simulink model "Sky_Sailor_Simulation"  (Simulink 8.3)
settings: Solver=ode3  StartTime=0.0  StopTime=20  FixedStep=0.05  RelTol=1e-3
libraries: simulink x1
settings Model: Creator=lestefan  LastModifiedBy=daniel
settings DataIOCC: ExternalInput=lw
settings OptimizationCC: ExpressionDepthLimit=2147483647  InitFltsAndDblsToZero=on
settings DebuggingCC: SaveWithParameterizedLinksMsg=none  SignalResolutionControl=TryResolveAllWithWarning  MultiTaskDSMMsg=warning  MultiTaskCondExecSysMsg=none  FcnCallInpInsideContextMsg=UseLocalSettings
settings SFSimCC: SimParseCustomCode=off
settings RTWCC: IncludeERTFirstTime=on
settings GRTTargetCC: TargetFcnLib=ansi_tfl_tmw.mat

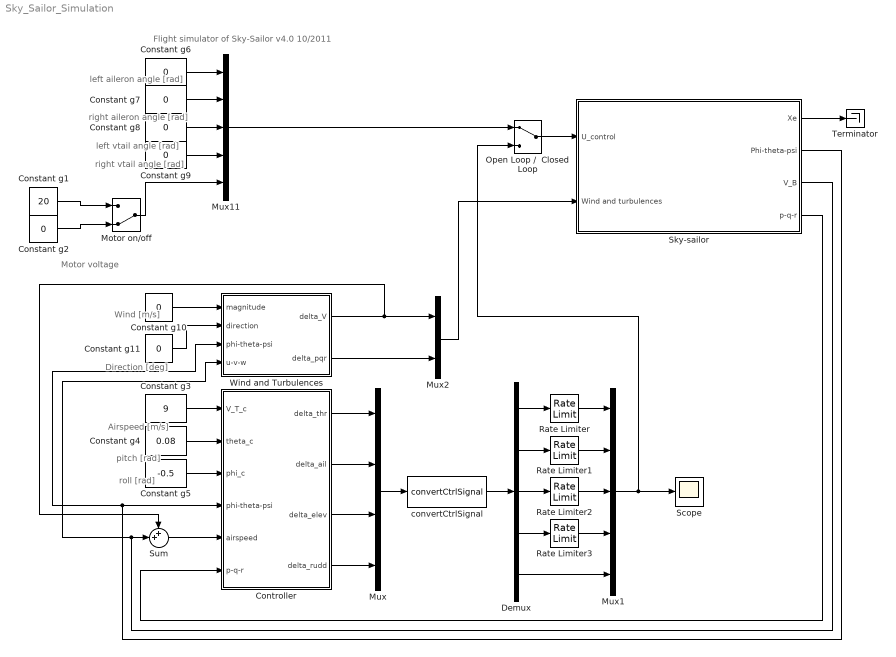
== system Sky_Sailor_Simulation ==
  note: Flight simulator of Sky-Sailor v4.0 10/2011
  note: left aileron angle [rad]
  note: right aileron angle [rad]
  note: left vtail angle [rad]
  note: right vtail angle [rad]
  note: Motor voltage
  note: Airspeed [m/s]
  note: pitch [rad]
  note: roll [rad]
  note: Wind [m/s]
  note: Direction [deg]
  Constant g1 : Constant  Value=20
  Constant g{2,6..11} (7 alike) : Constant  Value=0
  Constant g3 : Constant  Value=9
  Constant g4 : Constant  Value=0.08
  Constant g5 : Constant  Value=-0.5
  Controller : Subsystem
  Demux : Demux  Outputs=5
  Motor on/off : ManualSwitch  CurrentSetting=0
  Mux : Mux
  Mux1 : Mux  Inputs=5
  Mux11 : Mux  Inputs=5
  Mux2 : Mux  Inputs=2
  Open Loop /  Closed Loop : ManualSwitch
  Rate Limiter{,1..3} (4 alike) : RateLimiter  RisingSlewLimit=pi  FallingSlewLimit=-pi  SampleTimeMode=inherited
  Scope : Scope
      settings: YMin=-2.5  YMax=30  SaveName=ScopeData7
  Sky-sailor : Subsystem
  Sum : Sum  Inputs=++|
  Terminator : Terminator
  Wind and Turbulences : Subsystem
  convertCtrlSignal : MATLABFcn  MATLABFcn=convertCtrlSignal  OutputDimensions=5  OutputSignalType=real
  wires:
  Constant g6/1 -> Mux11/1
  Constant g7/1 -> Mux11/2
  Constant g8/1 -> Mux11/3
  Constant g9/1 -> Mux11/4
  Motor on/off/1 -> Mux11/5
  Sky-sailor/1(Xe) -> Terminator/1
  Constant g1/1 -> Motor on/off/1
  Constant g2/1 -> Motor on/off/2
  Constant g3/1 -> Controller/1(V_T_c)
  Constant g4/1 -> Controller/2(theta_c)
  Constant g5/1 -> Controller/3(phi_c)
  Mux11/1 -> Open Loop /  Closed Loop/1
  Open Loop /  Closed Loop/1 -> Sky-sailor/1(U_control)
  Mux1/1 -> Open Loop /  Closed Loop/2, Scope/1
  Sky-sailor/2(Phi-theta-psi) -> Controller/4(phi-theta-psi), Wind and Turbulences/3(phi-theta-psi)
  Sky-sailor/4(p-q-r) -> Controller/6(p-q-r)
  Controller/1(delta_thr) -> Mux/1
  Controller/2(delta_ail) -> Mux/2
  Controller/4(delta_rudd) -> Mux/4
  Demux/1 -> Rate Limiter/1
  Demux/2 -> Rate Limiter1/1
  Demux/3 -> Rate Limiter2/1
  Demux/4 -> Rate Limiter3/1
  Demux/5 -> Mux1/5
  Controller/3(delta_elev) -> Mux/3
  Rate Limiter/1 -> Mux1/1
  Rate Limiter1/1 -> Mux1/2
  Rate Limiter2/1 -> Mux1/3
  Rate Limiter3/1 -> Mux1/4
  Constant g10/1 -> Wind and Turbulences/1(magnitude)
  Sky-sailor/3(V_B) -> Sum/2, Wind and Turbulences/4(u-v-w)
  Sum/1 -> Controller/5(airspeed)
  Mux2/1 -> Sky-sailor/2(Wind and turbulences)
  Wind and Turbulences/1(delta_V) -> Mux2/1, Sum/1
  Wind and Turbulences/2(delta_pqr) -> Mux2/2
  Constant g11/1 -> Wind and Turbulences/2(direction)
  Mux/1 -> convertCtrlSignal/1
  convertCtrlSignal/1 -> Demux/1

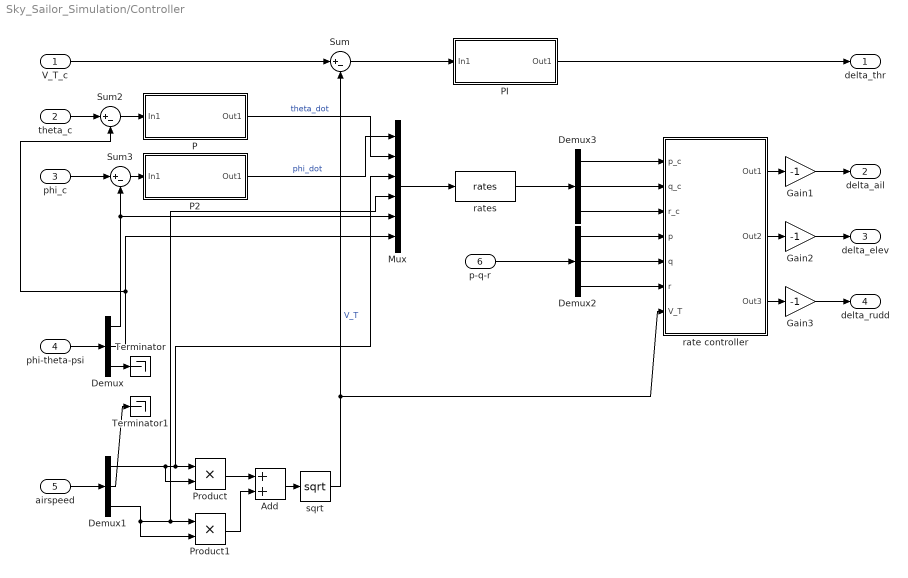
== system Sky_Sailor_Simulation/Controller ==
  V_T_c : Inport
  theta_c : Inport  Port=2
  phi_c : Inport  Port=3
  phi-theta-psi : Inport  Port=4
  airspeed : Inport  Port=5
  p-q-r : Inport  Port=6
  Add : Sum
  Demux{,1..3} (4 alike) : Demux  Outputs=3
  Gain1 : Gain  Gain=-1
  Gain2 : Gain  Gain=-1
  Gain3 : Gain  Gain=-1
  Mux : Mux  Inputs=6
  P : Subsystem
  P2 : Subsystem
  PI : Subsystem
  Product : Product  RndMeth=Zero
  Product1 : Product  RndMeth=Zero
  Sum : Sum  Inputs=|+-
  Sum2 : Sum  Inputs=|+-
  Sum3 : Sum  Inputs=|+-
  Terminator : Terminator
  Terminator1 : Terminator
  rate controller : Subsystem
  rates : MATLABFcn  MATLABFcn=rates  OutputDimensions=3  Output1D=off
  sqrt : Math  Operator=sqrt  SaturateOnIntegerOverflow=on
  delta_thr : Outport
  delta_ail : Outport  Port=2
  delta_elev : Outport  Port=3
  delta_rudd : Outport  Port=4
  wires:
  PI/1(Out1) -> delta_thr/1
  Gain1/1 -> delta_ail/1
  Gain2/1 -> delta_elev/1
  Gain3/1 -> delta_rudd/1
  phi-theta-psi/1 -> Demux/1
  airspeed/1 -> Demux1/1
  V_T_c/1 -> Sum/1
  Sum/1 -> PI/1(In1)
  Demux1/1 -> Product/1, Product/2, Mux/3
  Product/1 -> Add/1
  p-q-r/1 -> Demux2/1
  Product1/1 -> Add/2
  Add/1 -> sqrt/1
  sqrt/1 -> Sum/2, rate controller/7(V_T)  "V_T"
  Demux1/3 -> Product1/2, Product1/1, Mux/4
  Demux/1 -> Sum3/2, Mux/5
  Demux/2 -> Mux/6, Sum2/2
  theta_c/1 -> Sum2/1
  Sum2/1 -> P/1(In1)
  phi_c/1 -> Sum3/1
  Sum3/1 -> P2/1(In1)
  rate controller/1(Out1) -> Gain1/1
  rate controller/2(Out2) -> Gain2/1
  rate controller/3(Out3) -> Gain3/1
  Demux2/1 -> rate controller/4(p)
  Demux2/2 -> rate controller/5(q)
  Demux2/3 -> rate controller/6(r)
  Demux/3 -> Terminator/1
  Mux/1 -> rates/1
  P2/1(Out1) -> Mux/1  "phi_dot"
  P/1(Out1) -> Mux/2  "theta_dot"
  Demux1/2 -> Terminator1/1
  rates/1 -> Demux3/1
  Demux3/1 -> rate controller/1(p_c)
  Demux3/2 -> rate controller/2(q_c)
  Demux3/3 -> rate controller/3(r_c)

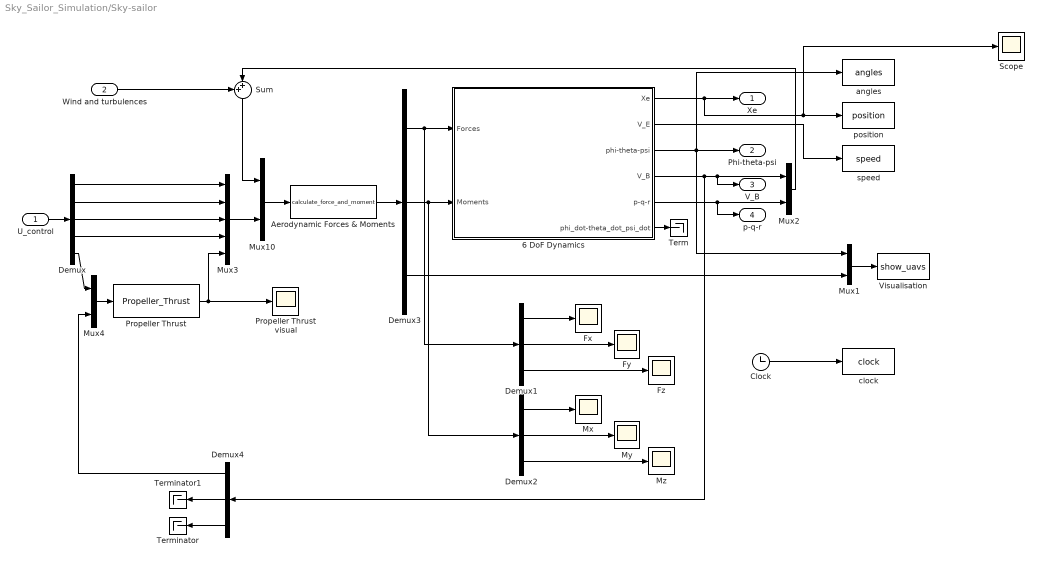
== system Sky_Sailor_Simulation/Sky-sailor ==
  U_control : Inport
  Wind and turbulences : Inport  Port=2
  "6 DoF Dynamics " : Subsystem
  Aerodynamic Forces & Moments : MATLABFcn  MATLABFcn=calculate_force_and_moment  OutputDimensions=7
  Clock : Clock
  Demux : Demux  Outputs=5
  Demux{1..4} (4 alike) : Demux  Outputs=3
  Fx : Scope
      settings: YMin=-0.58075  YMax=-0.57875
  Fy : Scope
      settings: YMin=-7e-016  YMax=4e-016
  Fz : Scope
      settings: YMin=-25.5725  YMax=-25.5325  SaveName=ScopeData2
  Mux{1..2,4,10} (4 alike) : Mux  Inputs=2
  Mux3 : Mux  Inputs=5
  Mx : Scope
      settings: YMin=-5e-015  YMax=5e-015  SaveName=ScopeData4
  My : Scope
      settings: YMin=-0.00025  YMax=0.0004  SaveName=ScopeData5
  Mz : Scope
      settings: YMin=-1.25e-016  YMax=1.75e-016  SaveName=ScopeData6
  Propeller Thrust : MATLABFcn  MATLABFcn=Propeller_Thrust  OutputDimensions=1
  Propeller Thrust visual : Scope
      settings: YMin=1.175  YMax=1.193  SaveName=ScopeData8
  Scope : Scope
      settings: SaveName=ScopeData3
  Sum : Sum  Inputs=++|
  Term : Terminator
  Terminator : Terminator
  Terminator1 : Terminator
  Visualisation : MATLABFcn  MATLABFcn=show_uavs  OutputDimensions=0
  angles : ToWorkspace  VariableName=angles  SampleTime=-1
  "clock " : ToWorkspace  VariableName=clock  SampleTime=-1
  position : ToWorkspace  VariableName=position  SampleTime=-1
  speed : ToWorkspace  VariableName=speed  SampleTime=-1
  Xe : Outport
  Phi-theta-psi : Outport  Port=2
  V_B : Outport  Port=3
  p-q-r : Outport  Port=4
  wires:
  "6 DoF Dynamics "/2(V_E) -> speed/1
  "6 DoF Dynamics "/3(phi-theta-psi) -> Phi-theta-psi/1, Mux1/1, angles/1
  "6 DoF Dynamics "/5(p-q-r) -> Mux2/2, p-q-r/1
  "6 DoF Dynamics "/4(V_B) -> Demux4/1, Mux2/1, V_B/1
  Demux3/1 -> "6 DoF Dynamics "/1(Forces), Demux1/1
  Demux3/2 -> "6 DoF Dynamics "/2(Moments), Demux2/1
  Aerodynamic Forces & Moments/1 -> Demux3/1
  Mux10/1 -> Aerodynamic Forces & Moments/1
  Mux1/1 -> Visualisation/1
  "6 DoF Dynamics "/1(Xe) -> Xe/1, position/1, Scope/1
  "6 DoF Dynamics "/6(phi_dot-theta_dot_psi_dot) -> Term/1
  Demux1/1 -> Fx/1
  Demux1/2 -> Fy/1
  Demux1/3 -> Fz/1
  Demux2/1 -> Mx/1
  Demux2/2 -> My/1
  Demux2/3 -> Mz/1
  U_control/1 -> Demux/1
  Demux/1 -> Mux3/1
  Demux/2 -> Mux3/2
  Demux/3 -> Mux3/3
  Demux/4 -> Mux3/4
  Mux3/1 -> Mux10/2
  Mux4/1 -> Propeller Thrust/1
  Demux/5 -> Mux4/1
  Demux4/3 -> Terminator/1
  Demux4/2 -> Terminator1/1
  Demux4/1 -> Mux4/2
  Propeller Thrust/1 -> Mux3/5, Propeller Thrust visual/1
  Demux3/3 -> Mux1/2
  Clock/1 -> "clock "/1
  Mux2/1 -> Sum/2
  Sum/1 -> Mux10/1
  Wind and turbulences/1 -> Sum/1

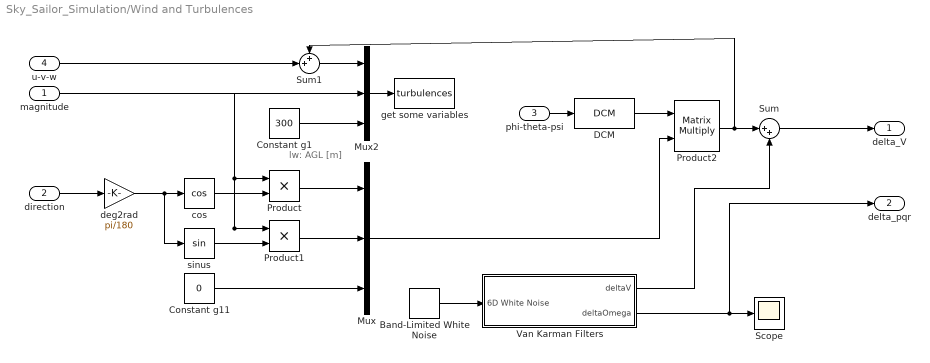
== system Sky_Sailor_Simulation/Wind and Turbulences ==
  note: lw: AGL [m]
  magnitude : Inport
  direction : Inport  Port=2
  phi-theta-psi : Inport  Port=3
  u-v-w : Inport  Port=4
  Band-Limited White Noise : simulink/Sources/Band-Limited White Noise  Cov=[1]  Ts=0.05  seed=[23341 23342 23343 23344 23345 23346]
  Constant g1 : Constant  Value=300
  Constant g11 : Constant  Value=0
  DCM : MATLABFcn  MATLABFcn=DCM  Output1D=off
  Mux : Mux  Inputs=3
  Mux2 : Mux  Inputs=3
  Product : Product  RndMeth=Zero
  Product1 : Product  RndMeth=Zero
  Product2 : Product  Multiplication=Matrix(*)  RndMeth=Zero
  Scope : Scope
      settings: YMin=-1  YMax=1  SaveName=ScopeData13
  Sum : Sum  Inputs=|++
  Sum1 : Sum  Inputs=++|
  Van Karman Filters : Subsystem
  cos : Trigonometry  Operator=cos
  deg2rad : Gain  Gain=pi/180
  get some variables : MATLABFcn  MATLABFcn=turbulences  OutputDimensions=0  Output1D=off
  sinus : Trigonometry
  delta_V : Outport
  delta_pqr : Outport  Port=2
  wires:
  direction/1 -> deg2rad/1
  deg2rad/1 -> cos/1, sinus/1
  cos/1 -> Product/2
  magnitude/1 -> Product/1, Product1/1, Mux2/2
  sinus/1 -> Product1/2
  Product1/1 -> Mux/2
  Product/1 -> Mux/1
  Constant g11/1 -> Mux/3
  phi-theta-psi/1 -> DCM/1
  Mux/1 -> Product2/2
  DCM/1 -> Product2/1
  Mux2/1 -> get some variables/1
  Band-Limited White Noise/1 -> Van Karman Filters/1(6D White Noise)
  Van Karman Filters/2(deltaOmega) -> delta_pqr/1, Scope/1
  Product2/1 -> Sum/1, Sum1/1
  Sum/1 -> delta_V/1
  Van Karman Filters/1(deltaV) -> Sum/2
  Constant g1/1 -> Mux2/3
  Sum1/1 -> Mux2/1
  u-v-w/1 -> Sum1/2

== system Sky_Sailor_Simulation/Controller/P ==
  In1 : Inport
  k_p : Gain  Gain=2
  Out1 : Outport
  wires:
  k_p/1 -> Out1/1
  In1/1 -> k_p/1

== system Sky_Sailor_Simulation/Controller/P2 ==
  In1 : Inport
  k_p : Gain  Gain=.2
  Out1 : Outport
  wires:
  k_p/1 -> Out1/1
  In1/1 -> k_p/1

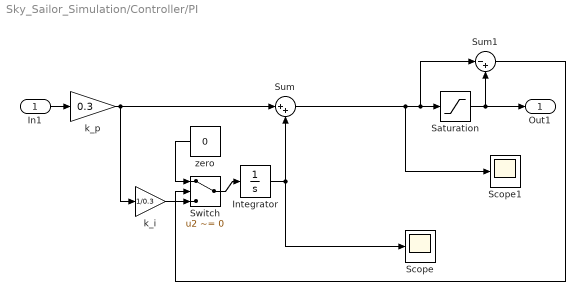
== system Sky_Sailor_Simulation/Controller/PI ==
  In1 : Inport
  Integrator : Integrator
  Saturation : Saturate  UpperLimit=1  LowerLimit=0  ZeroCross=off
  Scope : Scope
      settings: YMin=0.0927209  YMax=0.102481  SaveName=ScopeData11
  Scope1 : Scope
      settings: TimeRange=80  YMin=-0.4  YMax=1.1  SaveName=ScopeData12
  Sum : Sum  Inputs=|++
  Sum1 : Sum  Inputs=|-+
  Switch : Switch  Criteria=u2 ~= 0  ZeroCross=off
  k_i : Gain  Gain=1/0.3
  k_p : Gain  Gain=0.3
  zero : Constant  Value=0
  Out1 : Outport
  wires:
  In1/1 -> k_p/1
  Integrator/1 -> Sum/2, Scope/1
  k_p/1 -> Sum/1, k_i/1
  Saturation/1 -> Out1/1, Sum1/2
  Switch/1 -> Integrator/1
  Sum/1 -> Saturation/1, Sum1/1, Scope1/1
  Sum1/1 -> Switch/2
  k_i/1 -> Switch/3
  zero/1 -> Switch/1

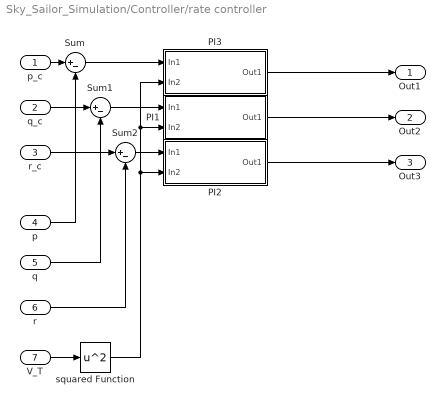
== system Sky_Sailor_Simulation/Controller/rate controller ==
  p_c : Inport
  q_c : Inport  Port=2
  r_c : Inport  Port=3
  p : Inport  Port=4
  q : Inport  Port=5
  r : Inport  Port=6
  V_T : Inport  Port=7
  PI1 : Subsystem
  PI2 : Subsystem
  PI3 : Subsystem
  Sum : Sum  Inputs=|+-
  Sum1 : Sum  Inputs=|+-
  Sum2 : Sum  Inputs=|+-
  squared Function : Math  Operator=square  SaturateOnIntegerOverflow=on
  Out1 : Outport
  Out2 : Outport  Port=2
  Out3 : Outport  Port=3
  wires:
  r_c/1 -> Sum2/1
  q_c/1 -> Sum1/1
  p_c/1 -> Sum/1
  p/1 -> Sum/2
  q/1 -> Sum1/2
  r/1 -> Sum2/2
  V_T/1 -> squared Function/1
  Sum1/1 -> PI1/1(In1)
  PI1/1(Out1) -> Out2/1
  Sum/1 -> PI3/1(In1)
  PI3/1(Out1) -> Out1/1
  PI2/1(Out1) -> Out3/1
  Sum2/1 -> PI2/1(In1)
  squared Function/1 -> PI3/2(In2), PI1/2(In2), PI2/2(In2)

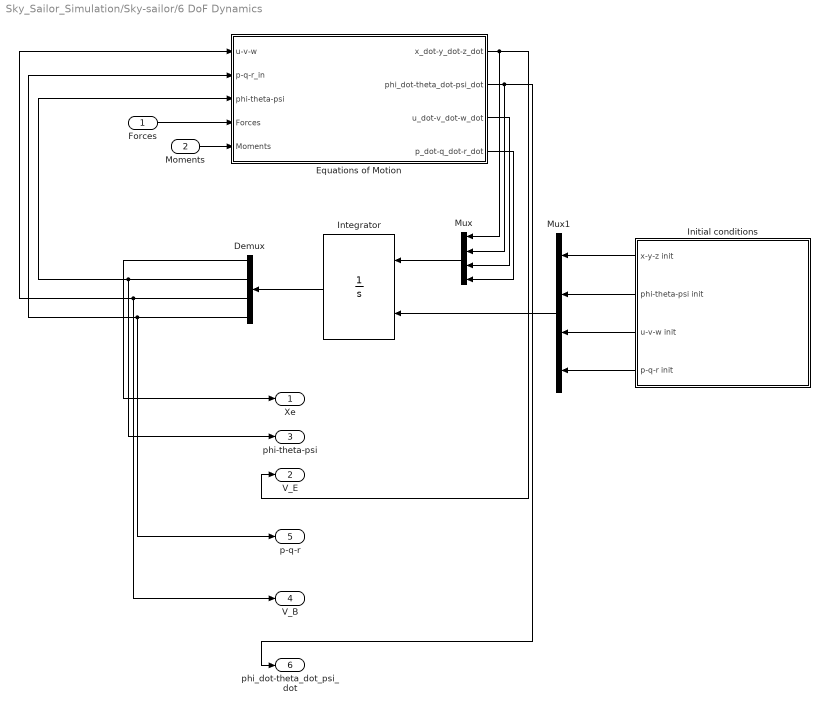
== system Sky_Sailor_Simulation/Sky-sailor/6 DoF Dynamics  ==
  Forces : Inport  PortDimensions=3
  Moments : Inport  Port=2  PortDimensions=3
  Demux : Demux
  Equations of Motion : Subsystem
  Initial conditions : Subsystem
  Integrator : Integrator  InitialConditionSource=external
  Mux : Mux
  Mux1 : Mux
  Xe : Outport
  V_E : Outport  Port=2
  phi-theta-psi : Outport  Port=3
  V_B : Outport  Port=4
  p-q-r : Outport  Port=5
  phi_dot-theta_dot_psi_dot : Outport  Port=6
  wires:
  Mux/1 -> Integrator/1
  Equations of Motion/1(x_dot-y_dot-z_dot) -> Mux/1, V_E/1
  Equations of Motion/2(phi_dot-theta_dot-psi_dot) -> Mux/2, phi_dot-theta_dot_psi_dot/1
  Equations of Motion/3(u_dot-v_dot-w_dot) -> Mux/3
  Equations of Motion/4(p_dot-q_dot-r_dot) -> Mux/4
  Mux1/1 -> Integrator/2
  Integrator/1 -> Demux/1
  Demux/1 -> Xe/1
  Demux/2 -> Equations of Motion/3(phi-theta-psi), phi-theta-psi/1
  Demux/3 -> Equations of Motion/1(u-v-w), V_B/1
  Demux/4 -> Equations of Motion/2(p-q-r_in), p-q-r/1
  Forces/1 -> Equations of Motion/4("Forces ")
  Moments/1 -> Equations of Motion/5(Moments)
  Initial conditions/1(x-y-z init) -> Mux1/1
  Initial conditions/2(phi-theta-psi init) -> Mux1/2
  Initial conditions/3(u-v-w init) -> Mux1/3
  Initial conditions/4(p-q-r init) -> Mux1/4

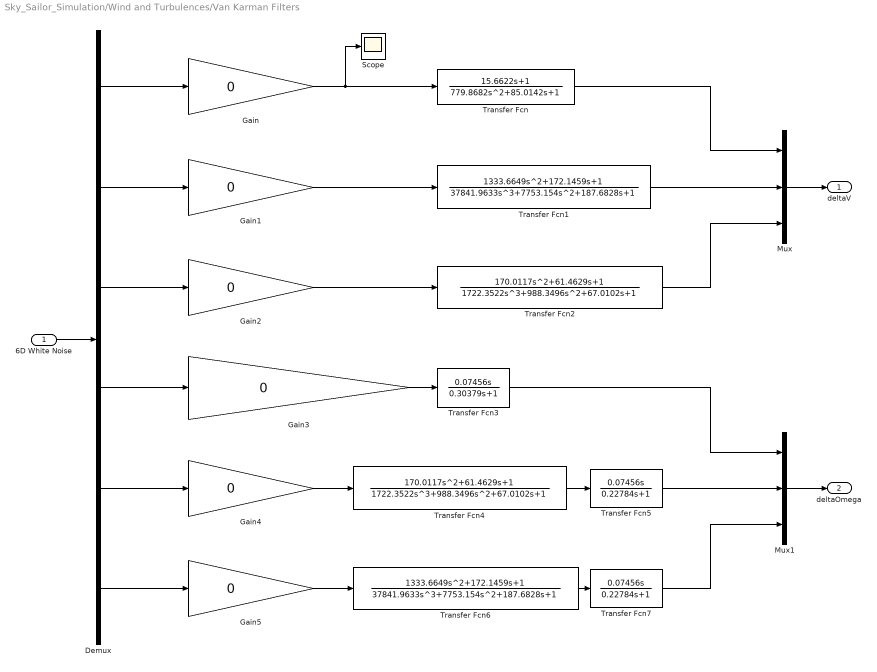
== system Sky_Sailor_Simulation/Wind and Turbulences/Van Karman Filters ==
  6D White Noise : Inport
  Demux : Demux  Outputs=6
  Gain{,1..5} (6 alike) : Gain  Gain=0
  Mux : Mux  Inputs=3
  Mux1 : Mux  Inputs=3
  Scope : Scope
      settings: YMin=-1  YMax=1  SaveName=ScopeData15
  Transfer Fcn : TransferFcn  Numerator=[15.6622 1]  Denominator=[779.8682 85.0142 1]
  Transfer Fcn1 : TransferFcn  Numerator=[1333.6649 172.1459 1]  Denominator=[37841.9633 7753.154 187.6828 1]
  Transfer Fcn2 : TransferFcn  Numerator=[170.0117 61.4629 1]  Denominator=[1722.3522 988.3496 67.0102 1]
  Transfer Fcn3 : TransferFcn  Numerator=[0.07456 0]  Denominator=[0.30379 1]
  Transfer Fcn4 : TransferFcn  Numerator=[170.0117 61.4629 1]  Denominator=[1722.3522 988.3496 67.0102 1]
  Transfer Fcn5 : TransferFcn  Numerator=[0.07456 0]  Denominator=[0.22784 1]
  Transfer Fcn6 : TransferFcn  Numerator=[1333.6649 172.1459 1]  Denominator=[37841.9633 7753.154 187.6828 1]
  Transfer Fcn7 : TransferFcn  Numerator=[0.07456 0]  Denominator=[0.22784 1]
  deltaV : Outport
  deltaOmega : Outport  Port=2
  wires:
  Transfer Fcn/1 -> Mux/1
  Gain/1 -> Transfer Fcn/1, Scope/1
  6D White Noise/1 -> Demux/1
  Mux/1 -> deltaV/1
  Mux1/1 -> deltaOmega/1
  Gain1/1 -> Transfer Fcn1/1
  Transfer Fcn1/1 -> Mux/2
  Gain2/1 -> Transfer Fcn2/1
  Transfer Fcn2/1 -> Mux/3
  Gain3/1 -> Transfer Fcn3/1
  Gain4/1 -> Transfer Fcn4/1
  Transfer Fcn4/1 -> Transfer Fcn5/1
  Transfer Fcn5/1 -> Mux1/2
  Transfer Fcn3/1 -> Mux1/1
  Gain5/1 -> Transfer Fcn6/1
  Transfer Fcn6/1 -> Transfer Fcn7/1
  Transfer Fcn7/1 -> Mux1/3
  Demux/1 -> Gain/1
  Demux/6 -> Gain5/1
  Demux/2 -> Gain1/1
  Demux/3 -> Gain2/1
  Demux/4 -> Gain3/1
  Demux/5 -> Gain4/1

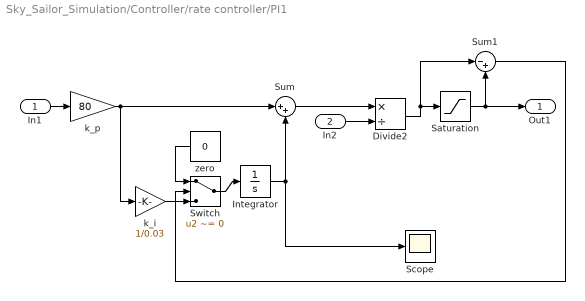
== system Sky_Sailor_Simulation/Controller/rate controller/PI1 ==
  In1 : Inport
  In2 : Inport  Port=2
  Divide2 : Product  Inputs=*/
  Integrator : Integrator
  Saturation : Saturate  UpperLimit=1  LowerLimit=-1  ZeroCross=off
  Scope : Scope
      settings: YMax=0.5  SaveName=ScopeData9
  Sum : Sum  Inputs=|++
  Sum1 : Sum  Inputs=|-+
  Switch : Switch  Criteria=u2 ~= 0  ZeroCross=off
  k_i : Gain  Gain=1/0.03
  k_p : Gain  Gain=80
  zero : Constant  Value=0
  Out1 : Outport
  wires:
  In1/1 -> k_p/1
  Integrator/1 -> Sum/2, Scope/1
  k_p/1 -> Sum/1, k_i/1
  Saturation/1 -> Out1/1, Sum1/2
  Switch/1 -> Integrator/1
  Sum/1 -> Divide2/1
  Divide2/1 -> Saturation/1, Sum1/1
  In2/1 -> Divide2/2
  Sum1/1 -> Switch/2
  zero/1 -> Switch/1
  k_i/1 -> Switch/3

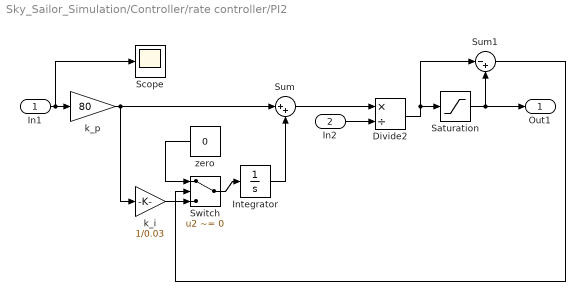
== system Sky_Sailor_Simulation/Controller/rate controller/PI2 ==
  In1 : Inport
  In2 : Inport  Port=2
  Divide2 : Product  Inputs=*/
  Integrator : Integrator
  Saturation : Saturate  UpperLimit=1  LowerLimit=-1  ZeroCross=off
  Scope : Scope
      settings: YMin=-0.075  YMax=0.125  SaveName=ScopeData10
  Sum : Sum  Inputs=|++
  Sum1 : Sum  Inputs=|-+
  Switch : Switch  Criteria=u2 ~= 0  ZeroCross=off
  k_i : Gain  Gain=1/0.03
  k_p : Gain  Gain=80
  zero : Constant  Value=0
  Out1 : Outport
  wires:
  Sum1/1 -> Switch/2
  In2/1 -> Divide2/2
  Divide2/1 -> Saturation/1, Sum1/1
  Sum/1 -> Divide2/1
  Switch/1 -> Integrator/1
  Saturation/1 -> Out1/1, Sum1/2
  k_p/1 -> Sum/1, k_i/1
  Integrator/1 -> Sum/2
  In1/1 -> k_p/1, Scope/1
  k_i/1 -> Switch/3
  zero/1 -> Switch/1

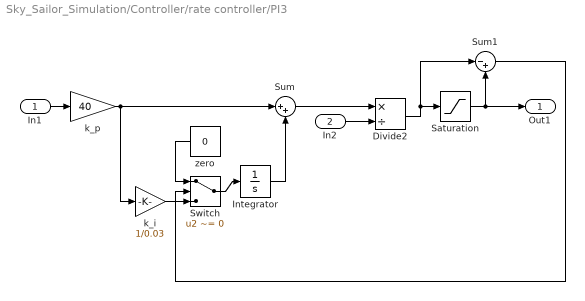
== system Sky_Sailor_Simulation/Controller/rate controller/PI3 ==
  In1 : Inport
  In2 : Inport  Port=2
  Divide2 : Product  Inputs=*/
  Integrator : Integrator
  Saturation : Saturate  UpperLimit=1  LowerLimit=-1  ZeroCross=off
  Sum : Sum  Inputs=|++
  Sum1 : Sum  Inputs=|-+
  Switch : Switch  Criteria=u2 ~= 0  ZeroCross=off
  k_i : Gain  Gain=1/0.03
  k_p : Gain  Gain=40
  zero : Constant  Value=0
  Out1 : Outport
  wires:
  In1/1 -> k_p/1
  Integrator/1 -> Sum/2
  k_p/1 -> Sum/1, k_i/1
  Saturation/1 -> Sum1/2, Out1/1
  Switch/1 -> Integrator/1
  Sum/1 -> Divide2/1
  Divide2/1 -> Saturation/1, Sum1/1
  In2/1 -> Divide2/2
  Sum1/1 -> Switch/2
  k_i/1 -> Switch/3
  zero/1 -> Switch/1

== system Sky_Sailor_Simulation/Sky-sailor/6 DoF Dynamics /Equations of Motion ==
  u-v-w : Inport
  p-q-r_in : Inport  Port=2
  phi-theta-psi : Inport  Port=3
  "Forces " : Inport  Port=4
  Moments : Inport  Port=5
  Demux : Demux
  Mux : Mux  Inputs=5
  eqn. of motion : MATLABFcn  MATLABFcn=dynamics  OutputDimensions=12
  x_dot-y_dot-z_dot : Outport
  phi_dot-theta_dot-psi_dot : Outport  Port=2
  u_dot-v_dot-w_dot : Outport  Port=3
  p_dot-q_dot-r_dot : Outport  Port=4
  wires:
  eqn. of motion/1 -> Demux/1
  Demux/1 -> x_dot-y_dot-z_dot/1
  Demux/2 -> phi_dot-theta_dot-psi_dot/1
  Demux/3 -> u_dot-v_dot-w_dot/1
  Demux/4 -> p_dot-q_dot-r_dot/1
  u-v-w/1 -> Mux/1
  p-q-r_in/1 -> Mux/2
  Moments/1 -> Mux/5
  "Forces "/1 -> Mux/4
  phi-theta-psi/1 -> Mux/3
  Mux/1 -> eqn. of motion/1

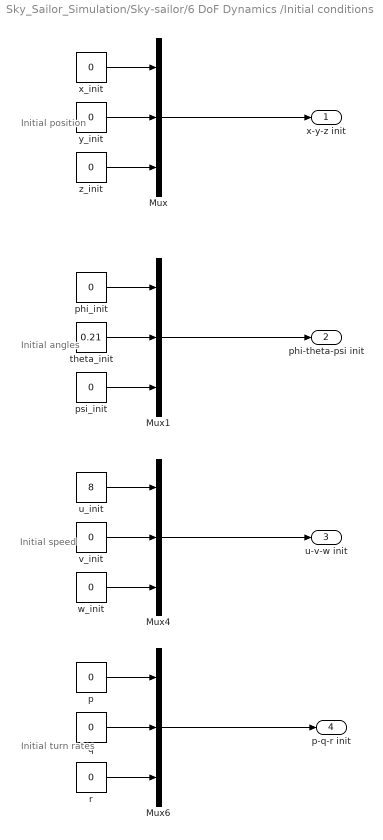
== system Sky_Sailor_Simulation/Sky-sailor/6 DoF Dynamics /Initial conditions ==
  note: Initial position
  note: Initial angles
  note: Initial turn rates
  note: Initial speed
  Mux{,1,4,6} (4 alike) : Mux  Inputs=3
  p : Constant  Value=0
  phi_init : Constant  Value=0
  psi_init : Constant  Value=0
  q : Constant  Value=0
  r : Constant  Value=0
  theta_init : Constant  Value=0.21
  u_init : Constant  Value=8
  v_init : Constant  Value=0
  w_init : Constant  Value=0
  x_init : Constant  Value=0
  y_init : Constant  Value=0
  z_init : Constant  Value=0
  x-y-z init : Outport
  phi-theta-psi init : Outport  Port=2
  u-v-w init : Outport  Port=3
  p-q-r init : Outport  Port=4
  wires:
  x_init/1 -> Mux/1
  y_init/1 -> Mux/2
  z_init/1 -> Mux/3
  phi_init/1 -> Mux1/1
  theta_init/1 -> Mux1/2
  psi_init/1 -> Mux1/3
  Mux/1 -> x-y-z init/1
  Mux1/1 -> phi-theta-psi init/1
  u_init/1 -> Mux4/1
  v_init/1 -> Mux4/2
  w_init/1 -> Mux4/3
  Mux4/1 -> u-v-w init/1
  p/1 -> Mux6/1
  q/1 -> Mux6/2
  r/1 -> Mux6/3
  Mux6/1 -> p-q-r init/1
